simulink model "SWC_HALOUT_type"  (R2021b)
settings: Solver=FixedStepDiscrete  StartTime=0.0  StopTime=10.0  FixedStep=0.001  RelTol=1e-3
values from neighbouring files (symbols this model uses):
  DIDLen_APPPedalZP = uint16(3)    [vcu_local_hdr.m]
  DIDLen_APSFunConfig = uint16(16)    [vcu_local_hdr.m]
  DIDLen_AutoLock = uint16(1)    [vcu_local_hdr.m]
  DIDLen_AutoWipHSpdEN = uint16(1)    [vcu_local_hdr.m]
  DIDLen_DKCKey = uint16(8)    [vcu_local_hdr.m]
  DIDLen_DRLDis = uint16(1)    [vcu_local_hdr.m]
  DIDLen_DynoMode = uint16(1)    [vcu_local_hdr.m]
  DIDLen_FMHTimer = uint16(1)    [vcu_local_hdr.m]
  DIDLen_LFLowPresThre = uint16(1)    [vcu_local_hdr.m]
  DIDLen_LFSensorID = uint16(4)    [vcu_local_hdr.m]
  DIDLen_LRLowPresThre = uint16(1)    [vcu_local_hdr.m]
  DIDLen_LRSensorID = uint16(4)    [vcu_local_hdr.m]
  DIDLen_NVMPedalZP = uint16(3)    [vcu_local_hdr.m]
  DIDLen_RFLowPresThre = uint16(1)    [vcu_local_hdr.m]
  DIDLen_RFSensorID = uint16(4)    [vcu_local_hdr.m]
  DIDLen_RRLowPresThre = uint16(1)    [vcu_local_hdr.m]
  DIDLen_RRSensorID = uint16(4)    [vcu_local_hdr.m]
  DIDLen_SensorMode = uint16(1)    [vcu_local_hdr.m]
  DIDLen_TireSize = uint16(16)    [vcu_local_hdr.m]
  DIDLen_TPMSLearnSta = uint16(1)    [vcu_local_hdr.m]
  DIDLen_TurnLampFLThreCurr = uint16(1)    [vcu_local_hdr.m]
  DIDLen_TurnLampFRThreCurr = uint16(1)    [vcu_local_hdr.m]
  DIDLen_TurnLampRLThreCurr = uint16(1)    [vcu_local_hdr.m]
  DIDLen_TurnLampRRThreCurr = uint16(1)    [vcu_local_hdr.m]
  DIDLen_USSConfig = uint16(16)    [vcu_local_hdr.m]
  DIDLen_WhlPres = uint16(4)    [vcu_local_hdr.m]
  DIDLen_WhlSensorBattSta = uint16(1)    [vcu_local_hdr.m]
  DIDLen_WhlTmp = uint16(4)    [vcu_local_hdr.m]
  DIDLen_WipRLSCmdCutFilter = uint16(1)    [vcu_local_hdr.m]
  DIDLen_WipRLSCmdHoldFilter = uint16(1)    [vcu_local_hdr.m]
  DIDLen_XWDMode = uint16(1)    [vcu_local_hdr.m]
  DIDNum_APPPedalZP = uint16(0x0206)    [vcu_local_hdr.m]
  DIDNum_APSFunConfig = uint16(0x0903)    [vcu_local_hdr.m]
  DIDNum_AutoLock = uint16(0x0306)    [vcu_local_hdr.m]
  DIDNum_AutoWipHSpdEN = uint16(0x0308)    [vcu_local_hdr.m]
  DIDNum_DKCKey = uint16(0x0202)    [vcu_local_hdr.m]
  DIDNum_DRLDis = uint16(0x0307)    [vcu_local_hdr.m]
  DIDNum_DynoMode = uint16(0x0203)    [vcu_local_hdr.m]
  DIDNum_FMHTimer = uint16(0x0305)    [vcu_local_hdr.m]
  DIDNum_LFLowPresThre = uint16(0x0B08)    [vcu_local_hdr.m]
  DIDNum_LFSensorID = uint16(0x0B01)    [vcu_local_hdr.m]
  DIDNum_LRLowPresThre = uint16(0x0B0A)    [vcu_local_hdr.m]
  DIDNum_LRSensorID = uint16(0x0B03)    [vcu_local_hdr.m]
  DIDNum_NVMPedalZP = uint16(0x0207)    [vcu_local_hdr.m]
  DIDNum_RFLowPresThre = uint16(0x0B09)    [vcu_local_hdr.m]
  DIDNum_RFSensorID = uint16(0x0B02)    [vcu_local_hdr.m]
  DIDNum_RRLowPresThre = uint16(0x0B0B)    [vcu_local_hdr.m]
  DIDNum_RRSensorID = uint16(0x0B04)    [vcu_local_hdr.m]
  DIDNum_SensorMode = uint16(0x0B0C)    [vcu_local_hdr.m]
  DIDNum_TireSize = uint16(0x0902)    [vcu_local_hdr.m]
  DIDNum_TPMSLearnSta = uint16(0x0B0D)    [vcu_local_hdr.m]
  DIDNum_TurnLampFLThreCurr = uint16(0x0303)    [vcu_local_hdr.m]
  DIDNum_TurnLampFRThreCurr = uint16(0x0301)    [vcu_local_hdr.m]
  DIDNum_TurnLampRLThreCurr = uint16(0x0304)    [vcu_local_hdr.m]
  DIDNum_TurnLampRRThreCurr = uint16(0x0302)    [vcu_local_hdr.m]
  DIDNum_USSConfig = uint16(0x0901)    [vcu_local_hdr.m]
  DIDNum_WhlPres = uint16(0x0B05)    [vcu_local_hdr.m]
  DIDNum_WhlSensorBattSta = uint16(0x0B07)    [vcu_local_hdr.m]
  DIDNum_WhlTmp = uint16(0x0B06)    [vcu_local_hdr.m]
  DIDNum_WipRLSCmdCutFilter = uint16(0x030A)    [vcu_local_hdr.m]
  DIDNum_WipRLSCmdHoldFilter = uint16(0x0309)    [vcu_local_hdr.m]
  DIDNum_XWDMode = uint16(0x0201)    [vcu_local_hdr.m]
  ENUM_TPMSLearnStatus_LEARNED = uint8(  1  )    [vcu_local_hdr.m]
  ENUM_TPMSLearnStatus_LEARNFAIL = uint8(  2  )    [vcu_local_hdr.m]
  ENUM_TPMSLearnStatus_NOTLEARN = uint8(  0  )    [vcu_local_hdr.m]
  FALSE = boolean( 0 )    [vcu_local_hdr.m]    (also in vcu_local_hdrTA2.m)
  TRUE = boolean( 1 )    [vcu_local_hdr.m]    (also in vcu_local_hdrTA2.m)
  ZERO_INT = uint8(0)    [vcu_local_hdr.m]    (also in vcu_local_hdrTA2.m)
undefined symbols (not defined in the file or in its folder): f32_ApsOutVehSpdSig, R_DIDWriteCDD_CSOP_DIDSet_APPPedalZP, R_DIDWriteCDD_CSOP_DIDSet_APSFunConfig, R_DIDWriteCDD_CSOP_DIDSet_AutoLock, R_DIDWriteCDD_CSOP_DIDSet_AutoWipHSpdEN, R_DIDWriteCDD_CSOP_DIDSet_DKCKey, R_DIDWriteCDD_CSOP_DIDSet_DRLDis, R_DIDWriteCDD_CSOP_DIDSet_DynoMode, R_DIDWriteCDD_CSOP_DIDSet_FMHTimer, R_DIDWriteCDD_CSOP_DIDSet_LFLowPresThre, R_DIDWriteCDD_CSOP_DIDSet_LFSensorID, R_DIDWriteCDD_CSOP_DIDSet_LRLowPresThre, R_DIDWriteCDD_CSOP_DIDSet_LRSensorID, R_DIDWriteCDD_CSOP_DIDSet_NVMPedalZP, R_DIDWriteCDD_CSOP_DIDSet_RFLowPresThre, R_DIDWriteCDD_CSOP_DIDSet_RFSensorID, R_DIDWriteCDD_CSOP_DIDSet_RRLowPresThre, R_DIDWriteCDD_CSOP_DIDSet_RRSensorID, R_DIDWriteCDD_CSOP_DIDSet_SensorMode, R_DIDWriteCDD_CSOP_DIDSet_TireSize, R_DIDWriteCDD_CSOP_DIDSet_TPMSLearnSta, R_DIDWriteCDD_CSOP_DIDSet_TurnLampFLThreCurr, R_DIDWriteCDD_CSOP_DIDSet_TurnLampFRThreCurr, R_DIDWriteCDD_CSOP_DIDSet_TurnLampRLThreCurr, R_DIDWriteCDD_CSOP_DIDSet_TurnLampRRThreCurr, R_DIDWriteCDD_CSOP_DIDSet_USSConfig, R_DIDWriteCDD_CSOP_DIDSet_WhlPres, R_DIDWriteCDD_CSOP_DIDSet_WhlSensorBattSta, R_DIDWriteCDD_CSOP_DIDSet_WhlTmp, R_DIDWriteCDD_CSOP_DIDSet_WipRLSCmdCutFilter, R_DIDWriteCDD_CSOP_DIDSet_WipRLSCmdHoldFilter, R_DIDWriteCDD_CSOP_DIDSet_XWDMode, R_FDCCDD_Inner_CSOP_FDC_AppCallSleep, R_HALINCDD_CSOP_PAS_Handler, R_HALINCDD_CSOP_UDS_Main, R_HALOUT_APS_CSOP_ApsOutput, R_HALOUTCDD_CSOP_AppNmStateReq, R_HALOUTCDD_CSOP_ResetPedalZeroPosDone, R_HALOUTCDD_CSOP_SetAcoreRebootCmdACK, R_HALOUTCDD_CSOP_SetHazardIND, R_HALOUTCDD_CSOP_SetSysPwrStat, R_HALOUTCDD_CSOP_SleepRequest, R_HALOUTCDD_CSOP_TPMSSensorIDRegSetResults, R_IOExpOUT_CDD_CSOP_IOExpSetVal, R_J1939_CAN1_FD1_CE100_0_CSOP_Write_CAN1_FD1_CE100_0, R_J1939_CAN1_FD1_CE100_1_CSOP_Write_CAN1_FD1_CE100_1, R_NVMWriteCDD_Inner_NVM_WriteOperation, R_UDSCDD_CSOP_DdmRestartOperationCycle, R_WDGCDD_CSOP_Call_WDG_AppEnd, u16_DIDLen_APPPedalZP, u16_DIDLen_APSFunConfig, u16_DIDLen_AutoLock, u16_DIDLen_AutoWipHSpdEN, u16_DIDLen_DKCKey, u16_DIDLen_DRLDis, u16_DIDLen_DynoMode, u16_DIDLen_FMHTimer, u16_DIDLen_LFLowPresThre, u16_DIDLen_LFSensorID, u16_DIDLen_LRLowPresThre ... (+95)
libraries: FVT_lib x142, simulink x107, hdlsllib x6, hcu_lib x5, halout x1
(part 1 of 8)
settings Model: DataDictionary=APPTypes.sldd  Creator=FVT23010  LastModifiedBy=FVT23010
settings DataIOCC: SaveFormat=StructureWithTime
settings OptimizationCC: DefaultParameterBehavior=Inlined  EnhancedBackFolding=on  PassReuseOutputArgsAs=Individual arguments  ZeroExternalMemoryAtStartup=off  ZeroInternalMemoryAtStartup=off  OptimizeBlockOrder=speed  DifferentSizesBufferReuse=on  OptimizationCustomize=off  EfficientTunableParamExpr=on
settings DebuggingCC: ParameterTunabilityLossMsg=error
settings ModelReferenceCC: ModelReferenceNumInstancesAllowed=Single
settings SFSimCC: MATLABDynamicMemAlloc=off
settings RTWCC: Description=AUTOSAR  SystemTargetFile=autosar.tlc  GenCodeOnly=on  TemplateMakefile=ert_default_tmf
settings CodeAppCC: ForceParamTrailComments=on  IgnoreCustomStorageClasses=off  OperatorAnnotations=on  SimulinkDataObjDesc=on  SFDataObjDesc=on  InsertBlockDesc=on
settings STFCustomTargetCC: TargetLangStandard=C99 (ISO)  MultiwordLength=256  ParMdlRefBuildCompliant=on  CompOptLevelCompliant=on  IncludeMdlTerminateFcn=off  CombineOutputUpdateFcns=on  SuppressErrorStatus=on  ERTCustomFileBanners=on  SupportNonFinite=off  SupportComplex=off  SupportContinuousTime=off  SupportNonInlinedSFcns=off  RemoveResetFunc=on  MATLABClassNameForMDSCustomization=Simulink.SoftwareTarget.ERTCustomization  AutosarCompliant=on  GRTInterface=off  UseToolchainInfoCompliant=on  LookupTableObjectStructAxisOrder=2,1,3,4,...  LUTObjectStructOrderEvenSpacing=Size,Table,Breakpoints  SystemTargetFile=autosar.tlc
settings ERTTargetCC: TargetLangStandard=C99 (ISO)  ConcurrentExecutionCompliant=off  IncludeMdlTerminateFcn=off  SuppressErrorStatus=on  SupportNonFinite=off  SupportComplex=off  ModelStepFunctionPrototypeControlCompliant=off  CPPClassGenCompliant=off  AutosarCompliant=on  LookupTableObjectStructAxisOrder=2,1,3,4,...  LUTObjectStructOrderEvenSpacing=Size,Table,Breakpoints  InlinedParameterPlacement=NonHierarchical  ERTCustomFileTemplate=example_file_process.tlc

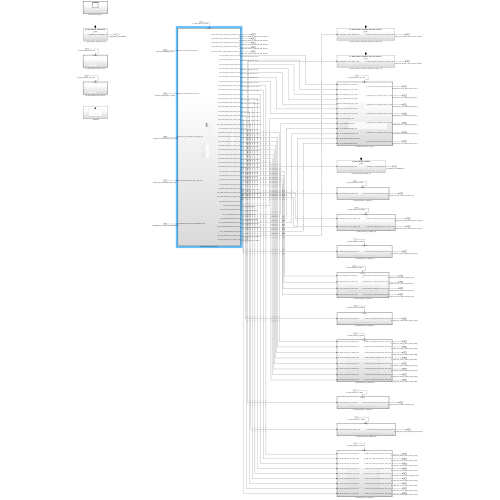
[thumbnail: Simulink's stored preview of the top-level diagram]
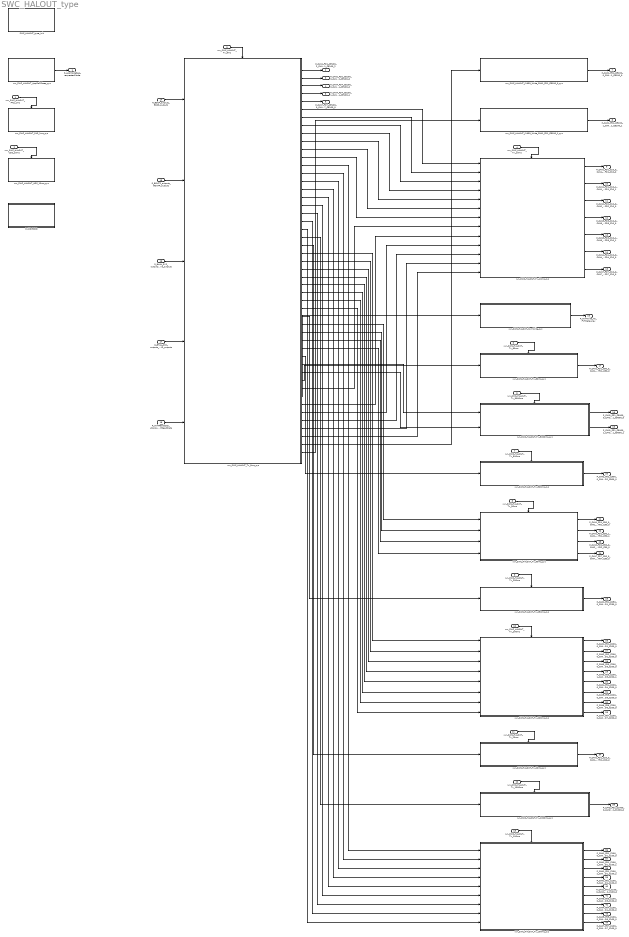
== system SWC_HALOUT_type ==
  run_SWC_HALOUT_PAS_1ms : Inport  SampleTime=0.001  OutputFunctionCall=on
  run_SWC_HALOUT_UDS_10ms : Inport  Port=2  SampleTime=0.01  OutputFunctionCall=on
  run_SWC_HALOUT_Tx_5ms : Inport  Port=3  SampleTime=0.005  OutputFunctionCall=on
  run_SWC_HALOUT_Tx_10ms : Inport  Port=4  SampleTime=0.01  OutputFunctionCall=on
  run_SWC_HALOUT_Tx_80ms : Inport  Port=5  SampleTime=0.08  OutputFunctionCall=on
  run_SWC_HALOUT_Tx_5000ms : Inport  Port=6  SampleTime=5  OutputFunctionCall=on
  run_SWC_HALOUT_Tx_500ms : Inport  Port=7  SampleTime=0.5  OutputFunctionCall=on
  run_SWC_HALOUT_Tx_50ms : Inport  Port=8  SampleTime=0.05  OutputFunctionCall=on
  run_SWC_HALOUT_Tx_250ms : Inport  Port=9  SampleTime=0.25  OutputFunctionCall=on
  run_SWC_HALOUT_Tx_200ms : Inport  Port=10  SampleTime=0.2  OutputFunctionCall=on
  run_SWC_HALOUT_Tx_20ms : Inport  Port=11  SampleTime=0.02  OutputFunctionCall=on
  run_SWC_HALOUT_Tx_1000ms : Inport  Port=12  SampleTime=1  OutputFunctionCall=on
  run_SWC_HALOUT_Tx_100ms : Inport  Port=13  SampleTime=0.1  OutputFunctionCall=on
  R_BSCP_outputs_BSCP_outputs : Inport  Port=14  OutDataTypeStr=Bus: BSCP_outputs  PortDimensions=1  BusOutputAsStruct=on
  R_BOUTP_outputs_BOUTP_outputs : Inport  Port=15  OutDataTypeStr=Bus: BOUTP_outputs  PortDimensions=1  BusOutputAsStruct=on
  R_BHAL_SYS_outputs_BHAL_SYS_outputs : Inport  Port=16  OutDataTypeStr=Bus: BHAL_SYS_outputs  PortDimensions=1  BusOutputAsStruct=on
  R_BHAL_DID_outputs_BHAL_DID_outputs : Inport  Port=17  OutDataTypeStr=Bus: BHAL_DID_outputs  PortDimensions=1  BusOutputAsStruct=on
  R_NVMReadCDD_u8Array1024_NVMReadData : Inport  Port=18  OutDataTypeStr=uint8  PortDimensions=1024
  P_WDGCDD : Subsystem
  SWC_HALOUT_type_Init : Subsystem
  run_SWC_HALOUT_AppCallSleep_sys : Subsystem
  run_SWC_HALOUT_J1939_Write_CAN1_FD1_CE100_0_sys : Subsystem
  run_SWC_HALOUT_J1939_Write_CAN1_FD1_CE100_1_sys : Subsystem
  run_SWC_HALOUT_NvmWrite_sys : Subsystem
  run_SWC_HALOUT_PAS_1ms_sys : Subsystem
  run_SWC_HALOUT_Tx_1000ms_sys : Subsystem
  run_SWC_HALOUT_Tx_100ms_sys : Subsystem
  run_SWC_HALOUT_Tx_10ms_sys : Subsystem
  run_SWC_HALOUT_Tx_200ms_sys : Subsystem
  run_SWC_HALOUT_Tx_20ms_sys : Subsystem
  run_SWC_HALOUT_Tx_250ms_sys : Subsystem
  run_SWC_HALOUT_Tx_5000ms_sys : Subsystem
  run_SWC_HALOUT_Tx_500ms_sys : Subsystem
  run_SWC_HALOUT_Tx_50ms_sys : Subsystem
  run_SWC_HALOUT_Tx_5ms_sys : Subsystem
  run_SWC_HALOUT_Tx_80ms_sys : Subsystem
  run_SWC_HALOUT_UDS_10ms_sys : Subsystem
  P_AppModeReq_requestedMode : Outport  OutDataTypeStr=Enum: AppModeRequestType  PortDimensions=1
  P_CAN1_FD1_CE100_2_CAN1_SG_FD1_CE100_2 : Outport  Port=2  OutDataTypeStr=Bus: DT_CAN1_SG_FD1_CE100_2  PortDimensions=1  BusOutputAsStruct=on
  P_CAN2_FD2_CE100_0_CAN2_SG_FD2_CE100_0 : Outport  Port=3  OutDataTypeStr=Bus: DT_CAN2_SG_FD2_CE100_0  PortDimensions=1  BusOutputAsStruct=on
  P_CAN4_FD4_CE100_0_CAN4_SG_FD4_CE100_0 : Outport  Port=4  OutDataTypeStr=Bus: DT_CAN4_SG_FD4_CE100_0  PortDimensions=1  BusOutputAsStruct=on
  P_CAN4_FD4_CE100_1_CAN4_SG_FD4_CE100_1 : Outport  Port=5  OutDataTypeStr=Bus: DT_CAN4_SG_FD4_CE100_1  PortDimensions=1  BusOutputAsStruct=on
  P_CAN7_FD7_CE100_0_CAN7_SG_FD7_CE100_0 : Outport  Port=6  OutDataTypeStr=Bus: DT_CAN7_SG_FD7_CE100_0  PortDimensions=1  BusOutputAsStruct=on
  P_CAN1_FD1_CE100_0_CAN1_SG_FD1_CE100_0 : Outport  Port=7  OutDataTypeStr=Bus: DT_CAN1_SG_FD1_CE100_0  PortDimensions=1  BusOutputAsStruct=on
  P_CAN1_FD1_CE100_1_CAN1_SG_FD1_CE100_1 : Outport  Port=8  OutDataTypeStr=Bus: DT_CAN1_SG_FD1_CE100_1  PortDimensions=1  BusOutputAsStruct=on
  P_CAN1_FD1_C10_0_CAN1_SG_FD1_C10_0 : Outport  Port=9  OutDataTypeStr=Bus: DT_CAN1_SG_FD1_C10_0  PortDimensions=1  BusOutputAsStruct=on
  P_CAN1_FD1_C10_1_CAN1_SG_FD1_C10_1 : Outport  Port=10  OutDataTypeStr=Bus: DT_CAN1_SG_FD1_C10_1  PortDimensions=1  BusOutputAsStruct=on
  P_CAN2_FD2_C10_0_CAN2_SG_FD2_C10_0 : Outport  Port=11  OutDataTypeStr=Bus: DT_CAN2_SG_FD2_C10_0  PortDimensions=1  BusOutputAsStruct=on
  P_CAN3_FD3_C10_0_CAN3_SG_FD3_C10_0 : Outport  Port=12  OutDataTypeStr=Bus: DT_CAN3_SG_FD3_C10_0  PortDimensions=1  BusOutputAsStruct=on
  P_CAN3_FD3_C10_1_CAN3_SG_FD3_C10_1 : Outport  Port=13  OutDataTypeStr=Bus: DT_CAN3_SG_FD3_C10_1  PortDimensions=1  BusOutputAsStruct=on
  P_CAN4_FD4_C10_0_CAN4_SG_FD4_C10_0 : Outport  Port=14  OutDataTypeStr=Bus: DT_CAN4_SG_FD4_C10_0  PortDimensions=1  BusOutputAsStruct=on
  P_CAN7_FD7_C10_0_CAN7_SG_FD7_C10_0 : Outport  Port=15  OutDataTypeStr=Bus: DT_CAN7_SG_FD7_C10_0  PortDimensions=1  BusOutputAsStruct=on
  P_NVMWrite_NV_FVTDataArray : Outport  Port=16  OutDataTypeStr=uint8  PortDimensions=1024
  P_CAN1_FD1_C80_0_CAN1_SG_FD1_C80_0 : Outport  Port=17  OutDataTypeStr=Bus: DT_CAN1_SG_FD1_C80_0  PortDimensions=1  BusOutputAsStruct=on
  P_CAN1_FD1_C5000_0_CAN1_SG_FD1_C5000_0 : Outport  Port=18  OutDataTypeStr=Bus: DT_CAN1_SG_FD1_C5000_0  PortDimensions=1  BusOutputAsStruct=on
  P_CAN1_FD1_C5000_1_CAN1_SG_FD1_C5000_1 : Outport  Port=19  OutDataTypeStr=Bus: DT_CAN1_SG_FD1_C5000_1  PortDimensions=1  BusOutputAsStruct=on
  P_CAN2_FD2_C500_0_CAN2_SG_FD2_C500_0 : Outport  Port=20  OutDataTypeStr=Bus: DT_CAN2_SG_FD2_C500_0  PortDimensions=1  BusOutputAsStruct=on
  P_CAN1_FD1_C50_0_CAN1_SG_FD1_C50_0 : Outport  Port=21  OutDataTypeStr=Bus: DT_CAN1_SG_FD1_C50_0  PortDimensions=1  BusOutputAsStruct=on
  P_CAN1_FD1_C50_1_CAN1_SG_FD1_C50_1 : Outport  Port=22  OutDataTypeStr=Bus: DT_CAN1_SG_FD1_C50_1  PortDimensions=1  BusOutputAsStruct=on
  P_CAN2_FD2_C50_0_CAN2_SG_FD2_C50_0 : Outport  Port=23  OutDataTypeStr=Bus: DT_CAN2_SG_FD2_C50_0  PortDimensions=1  BusOutputAsStruct=on
  P_CAN7_FD7_C50_0_CAN7_SG_FD7_C50_0 : Outport  Port=24  OutDataTypeStr=Bus: DT_CAN7_SG_FD7_C50_0  PortDimensions=1  BusOutputAsStruct=on
  P_CAN1_FD1_C250_0_CAN1_SG_FD1_C250_0 : Outport  Port=25  OutDataTypeStr=Bus: DT_CAN1_SG_FD1_C250_0  PortDimensions=1  BusOutputAsStruct=on
  P_CAN1_FD1_C200_0_CAN1_SG_FD1_C200_0 : Outport  Port=26  OutDataTypeStr=Bus: DT_CAN1_SG_FD1_C200_0  PortDimensions=1  BusOutputAsStruct=on
  P_CAN2_FD2_C200_0_CAN2_SG_FD2_C200_0 : Outport  Port=27  OutDataTypeStr=Bus: DT_CAN2_SG_FD2_C200_0  PortDimensions=1  BusOutputAsStruct=on
  P_CAN3_FD3_C200_0_CAN3_SG_FD3_C200_0 : Outport  Port=28  OutDataTypeStr=Bus: DT_CAN3_SG_FD3_C200_0  PortDimensions=1  BusOutputAsStruct=on
  P_CAN3_FD3_C200_1_CAN3_SG_FD3_C200_1 : Outport  Port=29  OutDataTypeStr=Bus: DT_CAN3_SG_FD3_C200_1  PortDimensions=1  BusOutputAsStruct=on
  P_CAN4_FD4_C200_0_CAN4_SG_FD4_C200_0 : Outport  Port=30  OutDataTypeStr=Bus: DT_CAN4_SG_FD4_C200_0  PortDimensions=1  BusOutputAsStruct=on
  P_CAN5_FD5_C200_0_CAN5_SG_FD5_C200_0 : Outport  Port=31  OutDataTypeStr=Bus: DT_CAN5_SG_FD5_C200_0  PortDimensions=1  BusOutputAsStruct=on
  P_CAN6_FD6_C200_0_CAN6_SG_FD6_C200_0 : Outport  Port=32  OutDataTypeStr=Bus: DT_CAN6_SG_FD6_C200_0  PortDimensions=1  BusOutputAsStruct=on
  P_CAN7_FD7_C200_0_CAN7_SG_FD7_C200_0 : Outport  Port=33  OutDataTypeStr=Bus: DT_CAN7_SG_FD7_C200_0  PortDimensions=1  BusOutputAsStruct=on
  P_CAN1_FD1_C20_0_CAN1_SG_FD1_C20_0 : Outport  Port=34  OutDataTypeStr=Bus: DT_CAN1_SG_FD1_C20_0  PortDimensions=1  BusOutputAsStruct=on
  P_CAN2_FD2_C1000_0_CAN2_SG_FD2_C1000_0 : Outport  Port=35  OutDataTypeStr=Bus: DT_CAN2_SG_FD2_C1000_0  PortDimensions=1  BusOutputAsStruct=on
  P_CAN1_FD1_C100_0_CAN1_SG_FD1_C100_0 : Outport  Port=36  OutDataTypeStr=Bus: DT_CAN1_SG_FD1_C100_0  PortDimensions=1  BusOutputAsStruct=on
  P_CAN1_FD1_C100_1_CAN1_SG_FD1_C100_1 : Outport  Port=37  OutDataTypeStr=Bus: DT_CAN1_SG_FD1_C100_1  PortDimensions=1  BusOutputAsStruct=on
  P_CAN1_FD1_C100_2_CAN1_SG_FD1_C100_2 : Outport  Port=38  OutDataTypeStr=Bus: DT_CAN1_SG_FD1_C100_2  PortDimensions=1  BusOutputAsStruct=on
  P_CAN1_FD1_C100_3_CAN1_SG_FD1_C100_3 : Outport  Port=39  OutDataTypeStr=Bus: DT_CAN1_SG_FD1_C100_3  PortDimensions=1  BusOutputAsStruct=on
  P_CAN2_GW2_C100_0_CAN2_SG_GW2_C100_0 : Outport  Port=40  OutDataTypeStr=Bus: DT_CAN2_SG_GW2_C100_0  PortDimensions=1  BusOutputAsStruct=on
  P_CAN3_FD3_C100_0_CAN3_SG_FD3_C100_0 : Outport  Port=41  OutDataTypeStr=Bus: DT_CAN3_SG_FD3_C100_0  PortDimensions=1  BusOutputAsStruct=on
  P_CAN4_FD4_C100_0_CAN4_SG_FD4_C100_0 : Outport  Port=42  OutDataTypeStr=Bus: DT_CAN4_SG_FD4_C100_0  PortDimensions=1  BusOutputAsStruct=on
  P_CAN5_FD5_C100_0_CAN5_SG_FD5_C100_0 : Outport  Port=43  OutDataTypeStr=Bus: DT_CAN5_SG_FD5_C100_0  PortDimensions=1  BusOutputAsStruct=on
  P_CAN7_FD7_C100_0_CAN7_SG_FD7_C100_0 : Outport  Port=44  OutDataTypeStr=Bus: DT_CAN7_SG_FD7_C100_0  PortDimensions=1  BusOutputAsStruct=on
  wires:
  run_SWC_HALOUT_AppCallSleep_sys/1(P_AppModeReq_requestedMode_write) -> P_AppModeReq_requestedMode/1
  R_BSCP_outputs_BSCP_outputs/1 -> run_SWC_HALOUT_Tx_5ms_sys/1(R_BSCP_outputs_BSCP_outputs_read)
  R_BOUTP_outputs_BOUTP_outputs/1 -> run_SWC_HALOUT_Tx_5ms_sys/2(R_BOUTP_outputs_BOUTP_outputs_read)
  R_BHAL_SYS_outputs_BHAL_SYS_outputs/1 -> run_SWC_HALOUT_Tx_5ms_sys/3(R_BHAL_SYS_outputs_BHAL_SYS_outputs_read)
  R_BHAL_DID_outputs_BHAL_DID_outputs/1 -> run_SWC_HALOUT_Tx_5ms_sys/4(R_BHAL_DID_outputs_BHAL_DID_outputs_read)
  R_NVMReadCDD_u8Array1024_NVMReadData/1 -> run_SWC_HALOUT_Tx_5ms_sys/5(R_NVMReadCDD_u8Array1024_NVMReadData_read)
  run_SWC_HALOUT_Tx_5ms_sys/1(P_CAN1_FD1_CE100_2_CAN1_SG_FD1_CE100_2_write) -> P_CAN1_FD1_CE100_2_CAN1_SG_FD1_CE100_2/1
  run_SWC_HALOUT_Tx_5ms_sys/2(P_CAN2_FD2_CE100_0_CAN2_SG_FD2_CE100_0_write) -> P_CAN2_FD2_CE100_0_CAN2_SG_FD2_CE100_0/1
  run_SWC_HALOUT_Tx_5ms_sys/3(P_CAN4_FD4_CE100_0_CAN4_SG_FD4_CE100_0_write) -> P_CAN4_FD4_CE100_0_CAN4_SG_FD4_CE100_0/1
  run_SWC_HALOUT_Tx_5ms_sys/4(P_CAN4_FD4_CE100_1_CAN4_SG_FD4_CE100_1_write) -> P_CAN4_FD4_CE100_1_CAN4_SG_FD4_CE100_1/1
  run_SWC_HALOUT_Tx_5ms_sys/5(P_CAN7_FD7_CE100_0_CAN7_SG_FD7_CE100_0_write) -> P_CAN7_FD7_CE100_0_CAN7_SG_FD7_CE100_0/1
  run_SWC_HALOUT_J1939_Write_CAN1_FD1_CE100_0_sys/1(P_CAN1_FD1_CE100_0_CAN1_SG_FD1_CE100_0_write) -> P_CAN1_FD1_CE100_0_CAN1_SG_FD1_CE100_0/1
  run_SWC_HALOUT_J1939_Write_CAN1_FD1_CE100_1_sys/1(P_CAN1_FD1_CE100_1_CAN1_SG_FD1_CE100_1_write) -> P_CAN1_FD1_CE100_1_CAN1_SG_FD1_CE100_1/1
  run_SWC_HALOUT_Tx_10ms_sys/1(P_CAN1_FD1_C10_0_CAN1_SG_FD1_C10_0_write) -> P_CAN1_FD1_C10_0_CAN1_SG_FD1_C10_0/1
  run_SWC_HALOUT_Tx_10ms_sys/2(P_CAN1_FD1_C10_1_CAN1_SG_FD1_C10_1_write) -> P_CAN1_FD1_C10_1_CAN1_SG_FD1_C10_1/1
  run_SWC_HALOUT_Tx_10ms_sys/3(P_CAN2_FD2_C10_0_CAN2_SG_FD2_C10_0_write) -> P_CAN2_FD2_C10_0_CAN2_SG_FD2_C10_0/1
  run_SWC_HALOUT_Tx_10ms_sys/4(P_CAN3_FD3_C10_0_CAN3_SG_FD3_C10_0_write) -> P_CAN3_FD3_C10_0_CAN3_SG_FD3_C10_0/1
  run_SWC_HALOUT_Tx_10ms_sys/5(P_CAN3_FD3_C10_1_CAN3_SG_FD3_C10_1_write) -> P_CAN3_FD3_C10_1_CAN3_SG_FD3_C10_1/1
  run_SWC_HALOUT_Tx_10ms_sys/6(P_CAN4_FD4_C10_0_CAN4_SG_FD4_C10_0_write) -> P_CAN4_FD4_C10_0_CAN4_SG_FD4_C10_0/1
  run_SWC_HALOUT_Tx_10ms_sys/7(P_CAN7_FD7_C10_0_CAN7_SG_FD7_C10_0_write) -> P_CAN7_FD7_C10_0_CAN7_SG_FD7_C10_0/1
  run_SWC_HALOUT_NvmWrite_sys/1(P_NVMWrite_NV_FVTDataArray_write) -> P_NVMWrite_NV_FVTDataArray/1
  run_SWC_HALOUT_Tx_80ms_sys/1(P_CAN1_FD1_C80_0_CAN1_SG_FD1_C80_0_write) -> P_CAN1_FD1_C80_0_CAN1_SG_FD1_C80_0/1
  run_SWC_HALOUT_Tx_5000ms_sys/1(P_CAN1_FD1_C5000_0_CAN1_SG_FD1_C5000_0_write) -> P_CAN1_FD1_C5000_0_CAN1_SG_FD1_C5000_0/1
  run_SWC_HALOUT_Tx_5000ms_sys/2(P_CAN1_FD1_C5000_1_CAN1_SG_FD1_C5000_1_write) -> P_CAN1_FD1_C5000_1_CAN1_SG_FD1_C5000_1/1
  run_SWC_HALOUT_Tx_500ms_sys/1(P_CAN2_FD2_C500_0_CAN2_SG_FD2_C500_0_write) -> P_CAN2_FD2_C500_0_CAN2_SG_FD2_C500_0/1
  run_SWC_HALOUT_Tx_50ms_sys/1(P_CAN1_FD1_C50_0_CAN1_SG_FD1_C50_0_write) -> P_CAN1_FD1_C50_0_CAN1_SG_FD1_C50_0/1
  run_SWC_HALOUT_Tx_50ms_sys/2(P_CAN1_FD1_C50_1_CAN1_SG_FD1_C50_1_write) -> P_CAN1_FD1_C50_1_CAN1_SG_FD1_C50_1/1
  run_SWC_HALOUT_Tx_50ms_sys/3(P_CAN2_FD2_C50_0_CAN2_SG_FD2_C50_0_write) -> P_CAN2_FD2_C50_0_CAN2_SG_FD2_C50_0/1
  run_SWC_HALOUT_Tx_50ms_sys/4(P_CAN7_FD7_C50_0_CAN7_SG_FD7_C50_0_write) -> P_CAN7_FD7_C50_0_CAN7_SG_FD7_C50_0/1
  run_SWC_HALOUT_Tx_250ms_sys/1(P_CAN1_FD1_C250_0_CAN1_SG_FD1_C250_0_write) -> P_CAN1_FD1_C250_0_CAN1_SG_FD1_C250_0/1
  run_SWC_HALOUT_Tx_200ms_sys/1(P_CAN1_FD1_C200_0_CAN1_SG_FD1_C200_0_write) -> P_CAN1_FD1_C200_0_CAN1_SG_FD1_C200_0/1
  run_SWC_HALOUT_Tx_200ms_sys/2(P_CAN2_FD2_C200_0_CAN2_SG_FD2_C200_0_write) -> P_CAN2_FD2_C200_0_CAN2_SG_FD2_C200_0/1
  run_SWC_HALOUT_Tx_200ms_sys/3(P_CAN3_FD3_C200_0_CAN3_SG_FD3_C200_0_write) -> P_CAN3_FD3_C200_0_CAN3_SG_FD3_C200_0/1
  run_SWC_HALOUT_Tx_200ms_sys/4(P_CAN3_FD3_C200_1_CAN3_SG_FD3_C200_1_write) -> P_CAN3_FD3_C200_1_CAN3_SG_FD3_C200_1/1
  run_SWC_HALOUT_Tx_200ms_sys/5(P_CAN4_FD4_C200_0_CAN4_SG_FD4_C200_0_write) -> P_CAN4_FD4_C200_0_CAN4_SG_FD4_C200_0/1
  run_SWC_HALOUT_Tx_200ms_sys/6(P_CAN5_FD5_C200_0_CAN5_SG_FD5_C200_0_write) -> P_CAN5_FD5_C200_0_CAN5_SG_FD5_C200_0/1
  run_SWC_HALOUT_Tx_200ms_sys/7(P_CAN6_FD6_C200_0_CAN6_SG_FD6_C200_0_write) -> P_CAN6_FD6_C200_0_CAN6_SG_FD6_C200_0/1
  run_SWC_HALOUT_Tx_200ms_sys/8(P_CAN7_FD7_C200_0_CAN7_SG_FD7_C200_0_write) -> P_CAN7_FD7_C200_0_CAN7_SG_FD7_C200_0/1
  run_SWC_HALOUT_Tx_20ms_sys/1(P_CAN1_FD1_C20_0_CAN1_SG_FD1_C20_0_write) -> P_CAN1_FD1_C20_0_CAN1_SG_FD1_C20_0/1
  run_SWC_HALOUT_Tx_1000ms_sys/1(P_CAN2_FD2_C1000_0_CAN2_SG_FD2_C1000_0_write) -> P_CAN2_FD2_C1000_0_CAN2_SG_FD2_C1000_0/1
  run_SWC_HALOUT_Tx_100ms_sys/1(P_CAN1_FD1_C100_0_CAN1_SG_FD1_C100_0_write) -> P_CAN1_FD1_C100_0_CAN1_SG_FD1_C100_0/1
  run_SWC_HALOUT_Tx_100ms_sys/2(P_CAN1_FD1_C100_1_CAN1_SG_FD1_C100_1_write) -> P_CAN1_FD1_C100_1_CAN1_SG_FD1_C100_1/1
  run_SWC_HALOUT_Tx_100ms_sys/3(P_CAN1_FD1_C100_2_CAN1_SG_FD1_C100_2_write) -> P_CAN1_FD1_C100_2_CAN1_SG_FD1_C100_2/1
  run_SWC_HALOUT_Tx_100ms_sys/4(P_CAN1_FD1_C100_3_CAN1_SG_FD1_C100_3_write) -> P_CAN1_FD1_C100_3_CAN1_SG_FD1_C100_3/1
  run_SWC_HALOUT_Tx_100ms_sys/5(P_CAN2_GW2_C100_0_CAN2_SG_GW2_C100_0_write) -> P_CAN2_GW2_C100_0_CAN2_SG_GW2_C100_0/1
  run_SWC_HALOUT_Tx_100ms_sys/6(P_CAN3_FD3_C100_0_CAN3_SG_FD3_C100_0_write) -> P_CAN3_FD3_C100_0_CAN3_SG_FD3_C100_0/1
  run_SWC_HALOUT_Tx_100ms_sys/7(P_CAN4_FD4_C100_0_CAN4_SG_FD4_C100_0_write) -> P_CAN4_FD4_C100_0_CAN4_SG_FD4_C100_0/1
  run_SWC_HALOUT_Tx_100ms_sys/8(P_CAN5_FD5_C100_0_CAN5_SG_FD5_C100_0_write) -> P_CAN5_FD5_C100_0_CAN5_SG_FD5_C100_0/1
  run_SWC_HALOUT_Tx_100ms_sys/9(P_CAN7_FD7_C100_0_CAN7_SG_FD7_C100_0_write) -> P_CAN7_FD7_C100_0_CAN7_SG_FD7_C100_0/1
  run_SWC_HALOUT_Tx_5ms_sys/6(IRV_ms10_CAN1_SG_FD1_C10_0_write) -> run_SWC_HALOUT_Tx_10ms_sys/1(IRV_ms10_CAN1_SG_FD1_C10_0_read)  "IRV_ms10_CAN1_SG_FD1_C10_0"
  run_SWC_HALOUT_Tx_5ms_sys/7(IRV_ms10_CAN1_SG_FD1_C10_1_write) -> run_SWC_HALOUT_Tx_10ms_sys/2(IRV_ms10_CAN1_SG_FD1_C10_1_read)  "IRV_ms10_CAN1_SG_FD1_C10_1"
  run_SWC_HALOUT_Tx_5ms_sys/8(IRV_ms10_CAN2_SG_FD2_C10_0_write) -> run_SWC_HALOUT_Tx_10ms_sys/3(IRV_ms10_CAN2_SG_FD2_C10_0_read)  "IRV_ms10_CAN2_SG_FD2_C10_0"
  run_SWC_HALOUT_Tx_5ms_sys/9(IRV_ms10_CAN3_SG_FD3_C10_0_write) -> run_SWC_HALOUT_Tx_10ms_sys/4(IRV_ms10_CAN3_SG_FD3_C10_0_read)  "IRV_ms10_CAN3_SG_FD3_C10_0"
  run_SWC_HALOUT_Tx_5ms_sys/10(IRV_ms10_CAN3_SG_FD3_C10_1_write) -> run_SWC_HALOUT_Tx_10ms_sys/5(IRV_ms10_CAN3_SG_FD3_C10_1_read)  "IRV_ms10_CAN3_SG_FD3_C10_1"
  run_SWC_HALOUT_Tx_5ms_sys/11(IRV_ms10_CAN4_SG_FD4_C10_0_write) -> run_SWC_HALOUT_Tx_10ms_sys/6(IRV_ms10_CAN4_SG_FD4_C10_0_read)  "IRV_ms10_CAN4_SG_FD4_C10_0"
  run_SWC_HALOUT_Tx_5ms_sys/12(IRV_ms10_CAN7_SG_FD7_C10_0_write) -> run_SWC_HALOUT_Tx_10ms_sys/7(IRV_ms10_CAN7_SG_FD7_C10_0_read)  "IRV_ms10_CAN7_SG_FD7_C10_0"
  run_SWC_HALOUT_Tx_5ms_sys/13(IRV_ms100_CAN1_SG_FD1_C100_0_write) -> run_SWC_HALOUT_Tx_100ms_sys/1(IRV_ms100_CAN1_SG_FD1_C100_0_read)  "IRV_ms100_CAN1_SG_FD1_C100_0"
  run_SWC_HALOUT_Tx_5ms_sys/14(IRV_ms100_CAN1_SG_FD1_C100_1_write) -> run_SWC_HALOUT_Tx_100ms_sys/2(IRV_ms100_CAN1_SG_FD1_C100_1_read)  "IRV_ms100_CAN1_SG_FD1_C100_1"
  run_SWC_HALOUT_Tx_5ms_sys/15(IRV_ms100_CAN1_SG_FD1_C100_2_write) -> run_SWC_HALOUT_Tx_100ms_sys/3(IRV_ms100_CAN1_SG_FD1_C100_2_read)  "IRV_ms100_CAN1_SG_FD1_C100_2"
  run_SWC_HALOUT_Tx_5ms_sys/16(IRV_ms100_CAN1_SG_FD1_C100_3_write) -> run_SWC_HALOUT_Tx_100ms_sys/4(IRV_ms100_CAN1_SG_FD1_C100_3_read)  "IRV_ms100_CAN1_SG_FD1_C100_3"
  run_SWC_HALOUT_Tx_5ms_sys/17(IRV_ms100_CAN2_SG_GW2_C100_0_write) -> run_SWC_HALOUT_Tx_100ms_sys/5(IRV_ms100_CAN2_SG_GW2_C100_0_read)  "IRV_ms100_CAN2_SG_GW2_C100_0"
  run_SWC_HALOUT_Tx_5ms_sys/18(IRV_ms100_CAN3_SG_FD3_C100_0_write) -> run_SWC_HALOUT_Tx_100ms_sys/6(IRV_ms100_CAN3_SG_FD3_C100_0_read)  "IRV_ms100_CAN3_SG_FD3_C100_0"
  run_SWC_HALOUT_Tx_5ms_sys/19(IRV_ms100_CAN4_SG_FD4_C100_0_write) -> run_SWC_HALOUT_Tx_100ms_sys/7(IRV_ms100_CAN4_SG_FD4_C100_0_read)  "IRV_ms100_CAN4_SG_FD4_C100_0"
  run_SWC_HALOUT_Tx_5ms_sys/20(IRV_ms100_CAN5_SG_FD5_C100_0_write) -> run_SWC_HALOUT_Tx_100ms_sys/8(IRV_ms100_CAN5_SG_FD5_C100_0_read)  "IRV_ms100_CAN5_SG_FD5_C100_0"
  run_SWC_HALOUT_Tx_5ms_sys/21(IRV_ms100_CAN7_SG_FD7_C100_0_write) -> run_SWC_HALOUT_Tx_100ms_sys/9(IRV_ms100_CAN7_SG_FD7_C100_0_read)  "IRV_ms100_CAN7_SG_FD7_C100_0"
  run_SWC_HALOUT_Tx_5ms_sys/22(IRV_ms1000_CAN2_SG_FD2_C1000_0_write) -> run_SWC_HALOUT_Tx_1000ms_sys/1(IRV_ms1000_CAN2_SG_FD2_C1000_0_read)  "IRV_ms1000_CAN2_SG_FD2_C1000_0"
  run_SWC_HALOUT_Tx_5ms_sys/23(IRV_ms20_CAN1_SG_FD1_C20_0_write) -> run_SWC_HALOUT_Tx_20ms_sys/1(IRV_ms20_CAN1_SG_FD1_C20_0_read)  "IRV_ms20_CAN1_SG_FD1_C20_0"
  run_SWC_HALOUT_Tx_5ms_sys/24(IRV_ms200_CAN1_SG_FD1_C200_0_write) -> run_SWC_HALOUT_Tx_200ms_sys/1(IRV_ms200_CAN1_SG_FD1_C200_0_read)  "IRV_ms200_CAN1_SG_FD1_C200_0"
  run_SWC_HALOUT_Tx_5ms_sys/25(IRV_ms200_CAN2_SG_FD2_C200_0_write) -> run_SWC_HALOUT_Tx_200ms_sys/2(IRV_ms200_CAN2_SG_FD2_C200_0_read)  "IRV_ms200_CAN2_SG_FD2_C200_0"
  run_SWC_HALOUT_Tx_5ms_sys/26(IRV_ms200_CAN3_SG_FD3_C200_0_write) -> run_SWC_HALOUT_Tx_200ms_sys/3(IRV_ms200_CAN3_SG_FD3_C200_0_read)  "IRV_ms200_CAN3_SG_FD3_C200_0"
  run_SWC_HALOUT_Tx_5ms_sys/27(IRV_ms200_CAN3_SG_FD3_C200_1_write) -> run_SWC_HALOUT_Tx_200ms_sys/4(IRV_ms200_CAN3_SG_FD3_C200_1_read)  "IRV_ms200_CAN3_SG_FD3_C200_1"
  run_SWC_HALOUT_Tx_5ms_sys/28(IRV_ms200_CAN4_SG_FD4_C200_0_write) -> run_SWC_HALOUT_Tx_200ms_sys/5(IRV_ms200_CAN4_SG_FD4_C200_0_read)  "IRV_ms200_CAN4_SG_FD4_C200_0"
  run_SWC_HALOUT_Tx_5ms_sys/29(IRV_ms200_CAN5_SG_FD5_C200_0_write) -> run_SWC_HALOUT_Tx_200ms_sys/6(IRV_ms200_CAN5_SG_FD5_C200_0_read)  "IRV_ms200_CAN5_SG_FD5_C200_0"
  run_SWC_HALOUT_Tx_5ms_sys/30(IRV_ms200_CAN6_SG_FD6_C200_0_write) -> run_SWC_HALOUT_Tx_200ms_sys/7(IRV_ms200_CAN6_SG_FD6_C200_0_read)  "IRV_ms200_CAN6_SG_FD6_C200_0"
  run_SWC_HALOUT_Tx_5ms_sys/31(IRV_ms200_CAN7_SG_FD7_C200_0_write) -> run_SWC_HALOUT_Tx_200ms_sys/8(IRV_ms200_CAN7_SG_FD7_C200_0_read)  "IRV_ms200_CAN7_SG_FD7_C200_0"
  run_SWC_HALOUT_Tx_5ms_sys/32(IRV_ms250_CAN1_SG_FD1_C250_0_write) -> run_SWC_HALOUT_Tx_250ms_sys/1(IRV_ms250_CAN1_SG_FD1_C250_0_read)  "IRV_ms250_CAN1_SG_FD1_C250_0"
  run_SWC_HALOUT_Tx_5ms_sys/33(IRV_ms50_CAN1_SG_FD1_C50_0_write) -> run_SWC_HALOUT_Tx_50ms_sys/1(IRV_ms50_CAN1_SG_FD1_C50_0_read)  "IRV_ms50_CAN1_SG_FD1_C50_0"
  run_SWC_HALOUT_Tx_5ms_sys/34(IRV_ms50_CAN1_SG_FD1_C50_1_write) -> run_SWC_HALOUT_Tx_50ms_sys/2(IRV_ms50_CAN1_SG_FD1_C50_1_read)  "IRV_ms50_CAN1_SG_FD1_C50_1"
  run_SWC_HALOUT_Tx_5ms_sys/35(IRV_ms50_CAN2_SG_FD2_C50_0_write) -> run_SWC_HALOUT_Tx_50ms_sys/3(IRV_ms50_CAN2_SG_FD2_C50_0_read)  "IRV_ms50_CAN2_SG_FD2_C50_0"
  run_SWC_HALOUT_Tx_5ms_sys/36(IRV_ms50_CAN7_SG_FD7_C50_0_write) -> run_SWC_HALOUT_Tx_50ms_sys/4(IRV_ms50_CAN7_SG_FD7_C50_0_read)  "IRV_ms50_CAN7_SG_FD7_C50_0"
  run_SWC_HALOUT_Tx_5ms_sys/37(IRV_ms500_CAN2_SG_FD2_C500_0_write) -> run_SWC_HALOUT_Tx_500ms_sys/1(IRV_ms500_CAN2_SG_FD2_C500_0_read)  "IRV_ms500_CAN2_SG_FD2_C500_0"
  run_SWC_HALOUT_Tx_5ms_sys/38(IRV_ms5000_CAN1_SG_FD1_C5000_0_write) -> run_SWC_HALOUT_Tx_5000ms_sys/1(IRV_ms5000_CAN1_SG_FD1_C5000_0_read)  "IRV_ms5000_CAN1_SG_FD1_C5000_0"
  run_SWC_HALOUT_Tx_5ms_sys/39(IRV_ms5000_CAN1_SG_FD1_C5000_1_write) -> run_SWC_HALOUT_Tx_5000ms_sys/2(IRV_ms5000_CAN1_SG_FD1_C5000_1_read)  "IRV_ms5000_CAN1_SG_FD1_C5000_1"
  run_SWC_HALOUT_Tx_5ms_sys/40(IRV_ms80_CAN1_SG_FD1_C80_0_write) -> run_SWC_HALOUT_Tx_80ms_sys/1(IRV_ms80_CAN1_SG_FD1_C80_0_read)  "IRV_ms80_CAN1_SG_FD1_C80_0"
  run_SWC_HALOUT_Tx_5ms_sys/41(IRV_f32_ApsOutVehSpdSig_write) -> run_SWC_HALOUT_Tx_10ms_sys/8(IRV_f32_ApsOutVehSpdSig_read)  "IRV_f32_ApsOutVehSpdSig"
  run_SWC_HALOUT_Tx_5ms_sys/42(IRV_u8Array1024_NvmWriteArray_write) -> run_SWC_HALOUT_NvmWrite_sys/1(IRV_u8Array1024_NvmWriteArray_read)  "IRV_u8Array1024_NvmWriteArray"
  run_SWC_HALOUT_Tx_5ms_sys/43(IRV_u8_ApsOutGearPosnSig_write) -> run_SWC_HALOUT_Tx_10ms_sys/9(IRV_u8_ApsOutGearPosnSig_read)  "IRV_u8_ApsOutGearPosnSig"
  run_SWC_HALOUT_Tx_5ms_sys/44(IRV_u8_ApsOutSendChrgPlugSta_write) -> run_SWC_HALOUT_Tx_10ms_sys/10(IRV_u8_ApsOutSendChrgPlugSta_read)  "IRV_u8_ApsOutSendChrgPlugSta"
  run_SWC_HALOUT_Tx_5ms_sys/45(IRV_u8_ApsOutSetFrSensorOnCmd_write) -> run_SWC_HALOUT_Tx_10ms_sys/11(IRV_u8_ApsOutSetFrSensorOnCmd_read)  "IRV_u8_ApsOutSetFrSensorOnCmd"
  run_SWC_HALOUT_Tx_5ms_sys/46(IRV_u8_ApsOutSetFrSensorSwTOCmd_write) -> run_SWC_HALOUT_Tx_10ms_sys/12(IRV_u8_ApsOutSetFrSensorSwTOCmd_read)  "IRV_u8_ApsOutSetFrSensorSwTOCmd"
  run_SWC_HALOUT_Tx_5ms_sys/47(IRV_u8_ApsOutSetVehSpdTOCmd_write) -> run_SWC_HALOUT_Tx_10ms_sys/13(IRV_u8_ApsOutSetVehSpdTOCmd_read)  "IRV_u8_ApsOutSetVehSpdTOCmd"
  run_SWC_HALOUT_Tx_5ms_sys/48(IRV_J1939_CAN1_SG_FD1_CE100_0_write) -> run_SWC_HALOUT_J1939_Write_CAN1_FD1_CE100_0_sys/1(IRV_J1939_CAN1_SG_FD1_CE100_0_read)  "IRV_J1939_CAN1_SG_FD1_CE100_0"
  run_SWC_HALOUT_Tx_5ms_sys/49(IRV_J1939_CAN1_SG_FD1_CE100_1_write) -> run_SWC_HALOUT_J1939_Write_CAN1_FD1_CE100_1_sys/1(IRV_J1939_CAN1_SG_FD1_CE100_1_read)  "IRV_J1939_CAN1_SG_FD1_CE100_1"
  run_SWC_HALOUT_PAS_1ms/1 -> run_SWC_HALOUT_PAS_1ms_sys/Trigger
  run_SWC_HALOUT_UDS_10ms/1 -> run_SWC_HALOUT_UDS_10ms_sys/Trigger
  run_SWC_HALOUT_Tx_5ms/1 -> run_SWC_HALOUT_Tx_5ms_sys/Trigger
  run_SWC_HALOUT_Tx_10ms/1 -> run_SWC_HALOUT_Tx_10ms_sys/Trigger
  run_SWC_HALOUT_Tx_80ms/1 -> run_SWC_HALOUT_Tx_80ms_sys/Trigger
  run_SWC_HALOUT_Tx_5000ms/1 -> run_SWC_HALOUT_Tx_5000ms_sys/Trigger
  run_SWC_HALOUT_Tx_500ms/1 -> run_SWC_HALOUT_Tx_500ms_sys/Trigger
  run_SWC_HALOUT_Tx_50ms/1 -> run_SWC_HALOUT_Tx_50ms_sys/Trigger
  run_SWC_HALOUT_Tx_250ms/1 -> run_SWC_HALOUT_Tx_250ms_sys/Trigger
  run_SWC_HALOUT_Tx_200ms/1 -> run_SWC_HALOUT_Tx_200ms_sys/Trigger
  run_SWC_HALOUT_Tx_20ms/1 -> run_SWC_HALOUT_Tx_20ms_sys/Trigger
  run_SWC_HALOUT_Tx_1000ms/1 -> run_SWC_HALOUT_Tx_1000ms_sys/Trigger
  run_SWC_HALOUT_Tx_100ms/1 -> run_SWC_HALOUT_Tx_100ms_sys/Trigger

== system SWC_HALOUT_type/P_WDGCDD ==
  run_SWC_HALOUT_AppCallWDG_End_sys : Subsystem

== system SWC_HALOUT_type/SWC_HALOUT_type_Init ==
  Event Listener : EventListener  EventName=reset

== system SWC_HALOUT_type/run_SWC_HALOUT_AppCallSleep_sys ==
  function : TriggerPort  TriggerType=function-call  IsSimulinkFunction=on  FunctionName=run_SWC_HALOUT_AppCallSleep  VariantControl=(inherit)
  Constant : Constant  Value=TRUE
  Data Type Conversion : DataTypeConversion  OutDataTypeStr=Enum: AppModeRequestType
  Data Type Conversion1 : DataTypeConversion  OutDataTypeStr=uint8
  P_AppModeReq_requestedMode_write : Outport
  wires:
  Data Type Conversion/1 -> P_AppModeReq_requestedMode_write/1
  Data Type Conversion1/1 -> Data Type Conversion/1
  Constant/1 -> Data Type Conversion1/1

== system SWC_HALOUT_type/run_SWC_HALOUT_J1939_Write_CAN1_FD1_CE100_0_sys ==
  IRV_J1939_CAN1_SG_FD1_CE100_0_read : Inport
  function : TriggerPort  TriggerType=function-call  IsSimulinkFunction=on  FunctionName=run_SWC_HALOUT_J1939_Write_CAN1_FD1_CE100_0  VariantControl=(inherit)
  P_CAN1_FD1_CE100_0_CAN1_SG_FD1_CE100_0_write : Outport
  wires:
  IRV_J1939_CAN1_SG_FD1_CE100_0_read/1 -> P_CAN1_FD1_CE100_0_CAN1_SG_FD1_CE100_0_write/1

== system SWC_HALOUT_type/run_SWC_HALOUT_J1939_Write_CAN1_FD1_CE100_1_sys ==
  IRV_J1939_CAN1_SG_FD1_CE100_1_read : Inport
  function : TriggerPort  TriggerType=function-call  IsSimulinkFunction=on  FunctionName=run_SWC_HALOUT_J1939_Write_CAN1_FD1_CE100_1  VariantControl=(inherit)
  P_CAN1_FD1_CE100_1_CAN1_SG_FD1_CE100_1_write : Outport
  wires:
  IRV_J1939_CAN1_SG_FD1_CE100_1_read/1 -> P_CAN1_FD1_CE100_1_CAN1_SG_FD1_CE100_1_write/1

== system SWC_HALOUT_type/run_SWC_HALOUT_NvmWrite_sys ==
  IRV_u8Array1024_NvmWriteArray_read : Inport
  function : TriggerPort  TriggerType=function-call  IsSimulinkFunction=on  FunctionName=run_SWC_HALOUT_NvmWrite  VariantControl=(inherit)
  P_NVMWrite_NV_FVTDataArray_write : Outport
  wires:
  IRV_u8Array1024_NvmWriteArray_read/1 -> P_NVMWrite_NV_FVTDataArray_write/1

== system SWC_HALOUT_type/run_SWC_HALOUT_PAS_1ms_sys ==
  function : TriggerPort  TriggerType=function-call  VariantControl=(inherit)  SampleTimeType=periodic  SampleTime=-1
  R_HALINCDD_CSOP_PAS_Handler : FunctionCaller  FunctionPrototype=R_HALINCDD_CSOP_PAS_Handler()

== system SWC_HALOUT_type/run_SWC_HALOUT_Tx_1000ms_sys ==
  IRV_ms1000_CAN2_SG_FD2_C1000_0_read : Inport
  function : TriggerPort  TriggerType=function-call  VariantControl=(inherit)  SampleTimeType=periodic  SampleTime=-1
  P_CAN2_FD2_C1000_0_CAN2_SG_FD2_C1000_0_write : Outport
  wires:
  IRV_ms1000_CAN2_SG_FD2_C1000_0_read/1 -> P_CAN2_FD2_C1000_0_CAN2_SG_FD2_C1000_0_write/1

== system SWC_HALOUT_type/run_SWC_HALOUT_Tx_100ms_sys ==
  IRV_ms100_CAN1_SG_FD1_C100_0_read : Inport
  IRV_ms100_CAN1_SG_FD1_C100_1_read : Inport  Port=2
  IRV_ms100_CAN1_SG_FD1_C100_2_read : Inport  Port=3
  IRV_ms100_CAN1_SG_FD1_C100_3_read : Inport  Port=4
  IRV_ms100_CAN2_SG_GW2_C100_0_read : Inport  Port=5
  IRV_ms100_CAN3_SG_FD3_C100_0_read : Inport  Port=6
  IRV_ms100_CAN4_SG_FD4_C100_0_read : Inport  Port=7
  IRV_ms100_CAN5_SG_FD5_C100_0_read : Inport  Port=8
  IRV_ms100_CAN7_SG_FD7_C100_0_read : Inport  Port=9
  function : TriggerPort  TriggerType=function-call  VariantControl=(inherit)  SampleTimeType=periodic  SampleTime=-1
  P_CAN1_FD1_C100_0_CAN1_SG_FD1_C100_0_write : Outport
  P_CAN1_FD1_C100_1_CAN1_SG_FD1_C100_1_write : Outport  Port=2
  P_CAN1_FD1_C100_2_CAN1_SG_FD1_C100_2_write : Outport  Port=3
  P_CAN1_FD1_C100_3_CAN1_SG_FD1_C100_3_write : Outport  Port=4
  P_CAN2_GW2_C100_0_CAN2_SG_GW2_C100_0_write : Outport  Port=5
  P_CAN3_FD3_C100_0_CAN3_SG_FD3_C100_0_write : Outport  Port=6
  P_CAN4_FD4_C100_0_CAN4_SG_FD4_C100_0_write : Outport  Port=7
  P_CAN5_FD5_C100_0_CAN5_SG_FD5_C100_0_write : Outport  Port=8
  P_CAN7_FD7_C100_0_CAN7_SG_FD7_C100_0_write : Outport  Port=9
  wires:
  IRV_ms100_CAN1_SG_FD1_C100_0_read/1 -> P_CAN1_FD1_C100_0_CAN1_SG_FD1_C100_0_write/1
  IRV_ms100_CAN1_SG_FD1_C100_1_read/1 -> P_CAN1_FD1_C100_1_CAN1_SG_FD1_C100_1_write/1
  IRV_ms100_CAN1_SG_FD1_C100_2_read/1 -> P_CAN1_FD1_C100_2_CAN1_SG_FD1_C100_2_write/1
  IRV_ms100_CAN1_SG_FD1_C100_3_read/1 -> P_CAN1_FD1_C100_3_CAN1_SG_FD1_C100_3_write/1
  IRV_ms100_CAN2_SG_GW2_C100_0_read/1 -> P_CAN2_GW2_C100_0_CAN2_SG_GW2_C100_0_write/1
  IRV_ms100_CAN3_SG_FD3_C100_0_read/1 -> P_CAN3_FD3_C100_0_CAN3_SG_FD3_C100_0_write/1
  IRV_ms100_CAN4_SG_FD4_C100_0_read/1 -> P_CAN4_FD4_C100_0_CAN4_SG_FD4_C100_0_write/1
  IRV_ms100_CAN5_SG_FD5_C100_0_read/1 -> P_CAN5_FD5_C100_0_CAN5_SG_FD5_C100_0_write/1
  IRV_ms100_CAN7_SG_FD7_C100_0_read/1 -> P_CAN7_FD7_C100_0_CAN7_SG_FD7_C100_0_write/1

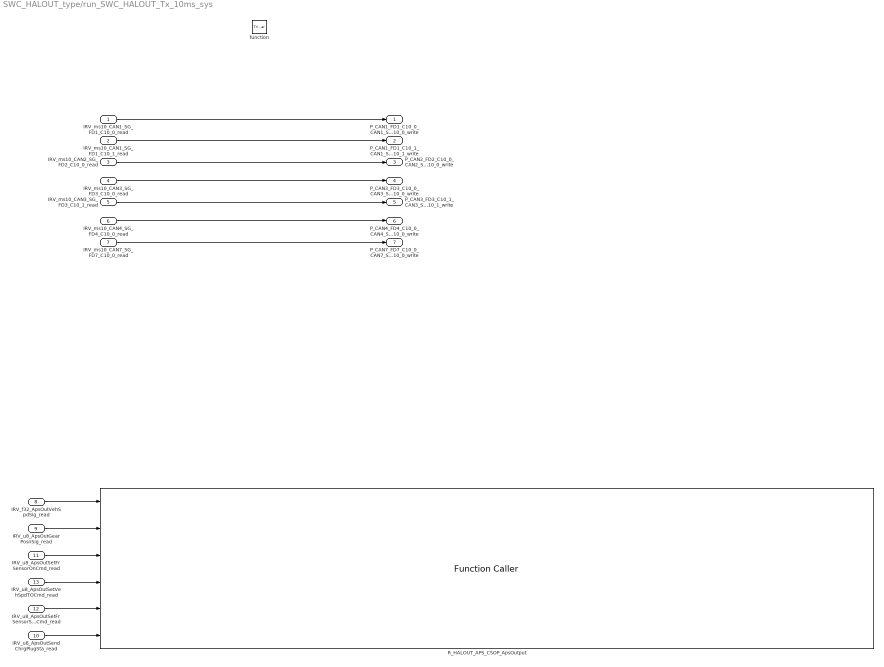
== system SWC_HALOUT_type/run_SWC_HALOUT_Tx_10ms_sys ==
  IRV_ms10_CAN1_SG_FD1_C10_0_read : Inport
  IRV_ms10_CAN1_SG_FD1_C10_1_read : Inport  Port=2
  IRV_ms10_CAN2_SG_FD2_C10_0_read : Inport  Port=3
  IRV_ms10_CAN3_SG_FD3_C10_0_read : Inport  Port=4
  IRV_ms10_CAN3_SG_FD3_C10_1_read : Inport  Port=5
  IRV_ms10_CAN4_SG_FD4_C10_0_read : Inport  Port=6
  IRV_ms10_CAN7_SG_FD7_C10_0_read : Inport  Port=7
  IRV_f32_ApsOutVehSpdSig_read : Inport  Port=8
  IRV_u8_ApsOutGearPosnSig_read : Inport  Port=9
  IRV_u8_ApsOutSendChrgPlugSta_read : Inport  Port=10
  IRV_u8_ApsOutSetFrSensorOnCmd_read : Inport  Port=11
  IRV_u8_ApsOutSetFrSensorSwTOCmd_read : Inport  Port=12
  IRV_u8_ApsOutSetVehSpdTOCmd_read : Inport  Port=13
  function : TriggerPort  TriggerType=function-call  VariantControl=(inherit)  SampleTimeType=periodic  SampleTime=-1
  R_HALOUT_APS_CSOP_ApsOutput : FunctionCaller  FunctionPrototype=R_HALOUT_APS_CSOP_ApsOutput(f32_ApsOutVehSpdSig,u8_ApsOutGearPosnSig,u8_ApsOutSetFrSensorOnCmd,u8_ApsOutSetVehSpdTOCmd,u8_ApsOutSetFrSensorSwTOCmd,u8_ApsOutSendChrgPlugSta)  InputArgumentSpecifications=single(1), uint8(1), uint8(1), uint8(1), uint8(1), uint8(1)
  P_CAN1_FD1_C10_0_CAN1_SG_FD1_C10_0_write : Outport
  P_CAN1_FD1_C10_1_CAN1_SG_FD1_C10_1_write : Outport  Port=2
  P_CAN2_FD2_C10_0_CAN2_SG_FD2_C10_0_write : Outport  Port=3
  P_CAN3_FD3_C10_0_CAN3_SG_FD3_C10_0_write : Outport  Port=4
  P_CAN3_FD3_C10_1_CAN3_SG_FD3_C10_1_write : Outport  Port=5
  P_CAN4_FD4_C10_0_CAN4_SG_FD4_C10_0_write : Outport  Port=6
  P_CAN7_FD7_C10_0_CAN7_SG_FD7_C10_0_write : Outport  Port=7
  wires:
  IRV_f32_ApsOutVehSpdSig_read/1 -> R_HALOUT_APS_CSOP_ApsOutput/1
  IRV_u8_ApsOutGearPosnSig_read/1 -> R_HALOUT_APS_CSOP_ApsOutput/2
  IRV_u8_ApsOutSetFrSensorOnCmd_read/1 -> R_HALOUT_APS_CSOP_ApsOutput/3
  IRV_u8_ApsOutSetVehSpdTOCmd_read/1 -> R_HALOUT_APS_CSOP_ApsOutput/4
  IRV_u8_ApsOutSetFrSensorSwTOCmd_read/1 -> R_HALOUT_APS_CSOP_ApsOutput/5
  IRV_u8_ApsOutSendChrgPlugSta_read/1 -> R_HALOUT_APS_CSOP_ApsOutput/6
  IRV_ms10_CAN1_SG_FD1_C10_0_read/1 -> P_CAN1_FD1_C10_0_CAN1_SG_FD1_C10_0_write/1
  IRV_ms10_CAN1_SG_FD1_C10_1_read/1 -> P_CAN1_FD1_C10_1_CAN1_SG_FD1_C10_1_write/1
  IRV_ms10_CAN2_SG_FD2_C10_0_read/1 -> P_CAN2_FD2_C10_0_CAN2_SG_FD2_C10_0_write/1
  IRV_ms10_CAN3_SG_FD3_C10_0_read/1 -> P_CAN3_FD3_C10_0_CAN3_SG_FD3_C10_0_write/1
  IRV_ms10_CAN3_SG_FD3_C10_1_read/1 -> P_CAN3_FD3_C10_1_CAN3_SG_FD3_C10_1_write/1
  IRV_ms10_CAN4_SG_FD4_C10_0_read/1 -> P_CAN4_FD4_C10_0_CAN4_SG_FD4_C10_0_write/1
  IRV_ms10_CAN7_SG_FD7_C10_0_read/1 -> P_CAN7_FD7_C10_0_CAN7_SG_FD7_C10_0_write/1

== system SWC_HALOUT_type/run_SWC_HALOUT_Tx_200ms_sys ==
  IRV_ms200_CAN1_SG_FD1_C200_0_read : Inport
  IRV_ms200_CAN2_SG_FD2_C200_0_read : Inport  Port=2
  IRV_ms200_CAN3_SG_FD3_C200_0_read : Inport  Port=3
  IRV_ms200_CAN3_SG_FD3_C200_1_read : Inport  Port=4
  IRV_ms200_CAN4_SG_FD4_C200_0_read : Inport  Port=5
  IRV_ms200_CAN5_SG_FD5_C200_0_read : Inport  Port=6
  IRV_ms200_CAN6_SG_FD6_C200_0_read : Inport  Port=7
  IRV_ms200_CAN7_SG_FD7_C200_0_read : Inport  Port=8
  function : TriggerPort  TriggerType=function-call  VariantControl=(inherit)  SampleTimeType=periodic  SampleTime=-1
  P_CAN1_FD1_C200_0_CAN1_SG_FD1_C200_0_write : Outport
  P_CAN2_FD2_C200_0_CAN2_SG_FD2_C200_0_write : Outport  Port=2
  P_CAN3_FD3_C200_0_CAN3_SG_FD3_C200_0_write : Outport  Port=3
  P_CAN3_FD3_C200_1_CAN3_SG_FD3_C200_1_write : Outport  Port=4
  P_CAN4_FD4_C200_0_CAN4_SG_FD4_C200_0_write : Outport  Port=5
  P_CAN5_FD5_C200_0_CAN5_SG_FD5_C200_0_write : Outport  Port=6
  P_CAN6_FD6_C200_0_CAN6_SG_FD6_C200_0_write : Outport  Port=7
  P_CAN7_FD7_C200_0_CAN7_SG_FD7_C200_0_write : Outport  Port=8
  wires:
  IRV_ms200_CAN1_SG_FD1_C200_0_read/1 -> P_CAN1_FD1_C200_0_CAN1_SG_FD1_C200_0_write/1
  IRV_ms200_CAN2_SG_FD2_C200_0_read/1 -> P_CAN2_FD2_C200_0_CAN2_SG_FD2_C200_0_write/1
  IRV_ms200_CAN3_SG_FD3_C200_0_read/1 -> P_CAN3_FD3_C200_0_CAN3_SG_FD3_C200_0_write/1
  IRV_ms200_CAN3_SG_FD3_C200_1_read/1 -> P_CAN3_FD3_C200_1_CAN3_SG_FD3_C200_1_write/1
  IRV_ms200_CAN4_SG_FD4_C200_0_read/1 -> P_CAN4_FD4_C200_0_CAN4_SG_FD4_C200_0_write/1
  IRV_ms200_CAN5_SG_FD5_C200_0_read/1 -> P_CAN5_FD5_C200_0_CAN5_SG_FD5_C200_0_write/1
  IRV_ms200_CAN6_SG_FD6_C200_0_read/1 -> P_CAN6_FD6_C200_0_CAN6_SG_FD6_C200_0_write/1
  IRV_ms200_CAN7_SG_FD7_C200_0_read/1 -> P_CAN7_FD7_C200_0_CAN7_SG_FD7_C200_0_write/1

== system SWC_HALOUT_type/run_SWC_HALOUT_Tx_20ms_sys ==
  IRV_ms20_CAN1_SG_FD1_C20_0_read : Inport
  function : TriggerPort  TriggerType=function-call  VariantControl=(inherit)  SampleTimeType=periodic  SampleTime=-1
  P_CAN1_FD1_C20_0_CAN1_SG_FD1_C20_0_write : Outport
  wires:
  IRV_ms20_CAN1_SG_FD1_C20_0_read/1 -> P_CAN1_FD1_C20_0_CAN1_SG_FD1_C20_0_write/1

== system SWC_HALOUT_type/run_SWC_HALOUT_Tx_250ms_sys ==
  IRV_ms250_CAN1_SG_FD1_C250_0_read : Inport
  function : TriggerPort  TriggerType=function-call  VariantControl=(inherit)  SampleTimeType=periodic  SampleTime=-1
  P_CAN1_FD1_C250_0_CAN1_SG_FD1_C250_0_write : Outport
  wires:
  IRV_ms250_CAN1_SG_FD1_C250_0_read/1 -> P_CAN1_FD1_C250_0_CAN1_SG_FD1_C250_0_write/1

== system SWC_HALOUT_type/run_SWC_HALOUT_Tx_5000ms_sys ==
  IRV_ms5000_CAN1_SG_FD1_C5000_0_read : Inport
  IRV_ms5000_CAN1_SG_FD1_C5000_1_read : Inport  Port=2
  function : TriggerPort  TriggerType=function-call  VariantControl=(inherit)  SampleTimeType=periodic  SampleTime=-1
  P_CAN1_FD1_C5000_0_CAN1_SG_FD1_C5000_0_write : Outport
  P_CAN1_FD1_C5000_1_CAN1_SG_FD1_C5000_1_write : Outport  Port=2
  wires:
  IRV_ms5000_CAN1_SG_FD1_C5000_0_read/1 -> P_CAN1_FD1_C5000_0_CAN1_SG_FD1_C5000_0_write/1
  IRV_ms5000_CAN1_SG_FD1_C5000_1_read/1 -> P_CAN1_FD1_C5000_1_CAN1_SG_FD1_C5000_1_write/1

== system SWC_HALOUT_type/run_SWC_HALOUT_Tx_500ms_sys ==
  IRV_ms500_CAN2_SG_FD2_C500_0_read : Inport
  function : TriggerPort  TriggerType=function-call  VariantControl=(inherit)  SampleTimeType=periodic  SampleTime=-1
  P_CAN2_FD2_C500_0_CAN2_SG_FD2_C500_0_write : Outport
  wires:
  IRV_ms500_CAN2_SG_FD2_C500_0_read/1 -> P_CAN2_FD2_C500_0_CAN2_SG_FD2_C500_0_write/1

== system SWC_HALOUT_type/run_SWC_HALOUT_Tx_50ms_sys ==
  IRV_ms50_CAN1_SG_FD1_C50_0_read : Inport
  IRV_ms50_CAN1_SG_FD1_C50_1_read : Inport  Port=2
  IRV_ms50_CAN2_SG_FD2_C50_0_read : Inport  Port=3
  IRV_ms50_CAN7_SG_FD7_C50_0_read : Inport  Port=4
  function : TriggerPort  TriggerType=function-call  VariantControl=(inherit)  SampleTimeType=periodic  SampleTime=-1
  P_CAN1_FD1_C50_0_CAN1_SG_FD1_C50_0_write : Outport
  P_CAN1_FD1_C50_1_CAN1_SG_FD1_C50_1_write : Outport  Port=2
  P_CAN2_FD2_C50_0_CAN2_SG_FD2_C50_0_write : Outport  Port=3
  P_CAN7_FD7_C50_0_CAN7_SG_FD7_C50_0_write : Outport  Port=4
  wires:
  IRV_ms50_CAN1_SG_FD1_C50_0_read/1 -> P_CAN1_FD1_C50_0_CAN1_SG_FD1_C50_0_write/1
  IRV_ms50_CAN1_SG_FD1_C50_1_read/1 -> P_CAN1_FD1_C50_1_CAN1_SG_FD1_C50_1_write/1
  IRV_ms50_CAN2_SG_FD2_C50_0_read/1 -> P_CAN2_FD2_C50_0_CAN2_SG_FD2_C50_0_write/1
  IRV_ms50_CAN7_SG_FD7_C50_0_read/1 -> P_CAN7_FD7_C50_0_CAN7_SG_FD7_C50_0_write/1
